simulink model "EPA_Walker"  (R2018a)
settings: Solver=FixedStepDiscrete  StartTime=0.0  StopTime=inf  FixedStep=0.001  RelTol=1e-3  EnableMultiTasking=on
model workspace (MAT data in the model file):
  MCOS : class17 (value not decoded)
undefined symbols (not defined in the file or in its folder): bits_current, bits_GRF, bits_Kd, bits_Kp, bits_position, bits_velocity, deadzone_in_TIB, deadzone_out_TIB, GRF_MAX, GRF_MIN, k_p_TIB, KD_MAX, KD_MIN, KP_MAX, KP_MIN, P_MAX, P_MIN, PressureFilter_CutOffFreq, PressureFilter_Gain, ReadingVoltage, T_MAX, T_MIN, V_MAX, V_MIN, voltageBias_GAS, voltageBias_GL, voltageBias_HAM, voltageBias_IL, voltageBias_POP, voltageBias_RF, voltageBias_SOL, voltageBias_TIB, voltageBias_VAS, voltageMultiplier_GAS, voltageMultiplier_GL, voltageMultiplier_HAM, voltageMultiplier_IL, voltageMultiplier_POP, voltageMultiplier_RF, voltageMultiplier_SOL, voltageMultiplier_TIB, voltageMultiplier_VAS, VoltageResolution
libraries: xpcethercatlib x139, simulink x19, peGeneralControl x18, slrtlib x9
(part 4 of 5)

== system EPA_Walker/PAMs/PAMs Right/IL ==
  Pressure Des : Inport
  Delay : Delay  DelayLength=1
  PID Controller : simulink/Continuous/PID Controller  Controller=PID  TimeDomain=Discrete-time  SampleTime=-1  IntegratorMethod=Forward Euler  FilterMethod=Forward Euler  Form=Ideal  UseFilter=on  ControllerParametersSource=external  P=k_p_pam  I=0  D=0.45*0.15/8  N=100  InitialConditionSource=internal  InitialConditionForIntegrator=0  InitialConditionForFilter=0  ExternalReset=none  LimitOutput=off  UpperSaturationLimit=inf  LowerSaturationLimit=-inf  LinearizeAsGain=on  AntiWindupMode=none  Kb=1  TrackingMode=off  Kt=1  PParamMin=[]  PParamMax=[]  IParamMin=[]  IParamMax=[]  DParamMin=[]  DParamMax=[]  NParamMin=[]  NParamMax=[]  KbParamMin=[]  KbParamMax=[]  KtParamMin=[]  KtParamMax=[]  POutMin=[]  POutMax=[]  IOutMin=[]  IOutMax=[]  DOutMin=[]  DOutMax=[]  NOutMin=[]  NOutMax=[]  KbOutMin=[]  KbOutMax=[]  KtOutMin=[]  KtOutMax=[]  IntegratorOutMin=[]  IntegratorOutMax=[]  FilterOutMin=[]  FilterOutMax=[]  SumOutMin=[]  SumOutMax=[]  SumI1OutMin=[]  SumI1OutMax=[]  SumI2OutMin=[]  SumI2OutMax=[]  SumI3OutMin=[]  SumI3OutMax=[]  SumDOutMin=[]  SumDOutMax=[]  SaturationOutMin=[]  SaturationOutMax=[]  IntegratorContinuousStateAttributes=''  IntegratorStateMustResolveToSignalObject=off  IntegratorRTWStateStorageClass=Auto  FilterContinuousStateAttributes=''  FilterStateMustResolveToSignalObject=off  FilterRTWStateStorageClass=Auto  DifferentiatorICPrevScaledInput=0  DifferentiatorOutMin=[]  DifferentiatorOutMax=[]  FilterDiffOutCoefMin=[]  FilterDiffOutCoefMax=[]  SumDenOutMin=[]  SumDenOutMax=[]  SumNumOutMin=[]  SumNumOutMax=[]  ReciprocalOutMin=[]  ReciprocalOutMax=[]  DivideOutMin=[]  DivideOutMax=[]  TunerSelectOption=Transfer Function Based (PID Tuner App)
  Solenoids : MATLAB Function  TreatAsAtomicUnit=on
  Sum : Sum  Inputs=|+-
  tag scope: R_IL_in=global, R_IL_out=global
  wires:
  Solenoids/3(inside_deadzone_1) -> Delay/1
  Delay/1 -> Solenoids/2(inside_deadzone)
  Pressure Des/1 -> Sum/1
  [R_IL_pres] -> Sum/2
  [R_deadzone_in] -> Solenoids/3(deadzone_in)
  [R_deadzone_out] -> Solenoids/4(deadzone_out)
  Solenoids/1(intake) -> [R_IL_in]
  Solenoids/2(outtake) -> [R_IL_out]
  [R_k_i] -> PID Controller/3
  [R_k_d] -> PID Controller/4
  [R_N] -> PID Controller/5
  Sum/1 -> PID Controller/1
  PID Controller/1 -> Solenoids/1(control)
  [R_k_p] -> PID Controller/2
  [R_PAMs_off] -> Solenoids/5(PAMs_on)
  [System_on] -> Solenoids/6(System_on)
  [R_Depressurize_PAMs] -> Solenoids/7(depressurize)

== system EPA_Walker/PAMs/PAMs Right/POP ==
  Pressure Des : Inport
  Delay : Delay  DelayLength=1
  PID Controller : simulink/Continuous/PID Controller  Controller=PID  TimeDomain=Discrete-time  SampleTime=-1  IntegratorMethod=Forward Euler  FilterMethod=Forward Euler  Form=Ideal  UseFilter=on  ControllerParametersSource=external  P=k_p_pam  I=0  D=0.45*0.15/8  N=100  InitialConditionSource=internal  InitialConditionForIntegrator=0  InitialConditionForFilter=0  ExternalReset=none  LimitOutput=off  UpperSaturationLimit=inf  LowerSaturationLimit=-inf  LinearizeAsGain=on  AntiWindupMode=none  Kb=1  TrackingMode=off  Kt=1  PParamMin=[]  PParamMax=[]  IParamMin=[]  IParamMax=[]  DParamMin=[]  DParamMax=[]  NParamMin=[]  NParamMax=[]  KbParamMin=[]  KbParamMax=[]  KtParamMin=[]  KtParamMax=[]  POutMin=[]  POutMax=[]  IOutMin=[]  IOutMax=[]  DOutMin=[]  DOutMax=[]  NOutMin=[]  NOutMax=[]  KbOutMin=[]  KbOutMax=[]  KtOutMin=[]  KtOutMax=[]  IntegratorOutMin=[]  IntegratorOutMax=[]  FilterOutMin=[]  FilterOutMax=[]  SumOutMin=[]  SumOutMax=[]  SumI1OutMin=[]  SumI1OutMax=[]  SumI2OutMin=[]  SumI2OutMax=[]  SumI3OutMin=[]  SumI3OutMax=[]  SumDOutMin=[]  SumDOutMax=[]  SaturationOutMin=[]  SaturationOutMax=[]  IntegratorContinuousStateAttributes=''  IntegratorStateMustResolveToSignalObject=off  IntegratorRTWStateStorageClass=Auto  FilterContinuousStateAttributes=''  FilterStateMustResolveToSignalObject=off  FilterRTWStateStorageClass=Auto  DifferentiatorICPrevScaledInput=0  DifferentiatorOutMin=[]  DifferentiatorOutMax=[]  FilterDiffOutCoefMin=[]  FilterDiffOutCoefMax=[]  SumDenOutMin=[]  SumDenOutMax=[]  SumNumOutMin=[]  SumNumOutMax=[]  ReciprocalOutMin=[]  ReciprocalOutMax=[]  DivideOutMin=[]  DivideOutMax=[]  TunerSelectOption=Transfer Function Based (PID Tuner App)
  Solenoids : MATLAB Function  TreatAsAtomicUnit=on
  Sum : Sum  Inputs=|+-
  tag scope: R_POP_in=global, R_POP_out=global
  wires:
  Solenoids/3(inside_deadzone_1) -> Delay/1
  Delay/1 -> Solenoids/2(inside_deadzone)
  Pressure Des/1 -> Sum/1
  [R_POP_pres] -> Sum/2
  [R_deadzone_in_pop] -> Solenoids/3(deadzone_in)
  [R_deadzone_out_pop] -> Solenoids/4(deadzone_out)
  Solenoids/1(intake) -> [R_POP_in]
  Solenoids/2(outtake) -> [R_POP_out]
  [R_k_i] -> PID Controller/3
  [R_k_d] -> PID Controller/4
  [R_N] -> PID Controller/5
  Sum/1 -> PID Controller/1
  PID Controller/1 -> Solenoids/1(control)
  [R_k_p] -> PID Controller/2
  [R_PAMs_off] -> Solenoids/5(PAMs_on)
  [System_on] -> Solenoids/6(System_on)
  [R_Depressurize_PAMs] -> Solenoids/7(depressurize)

== system EPA_Walker/PAMs/PAMs Right/RF ==
  Pressure Des : Inport
  Delay : Delay  DelayLength=1
  PID Controller : simulink/Continuous/PID Controller  Controller=PID  TimeDomain=Discrete-time  SampleTime=-1  IntegratorMethod=Forward Euler  FilterMethod=Forward Euler  Form=Ideal  UseFilter=on  ControllerParametersSource=external  P=k_p_pam  I=0  D=0.45*0.15/8  N=100  InitialConditionSource=internal  InitialConditionForIntegrator=0  InitialConditionForFilter=0  ExternalReset=none  LimitOutput=off  UpperSaturationLimit=inf  LowerSaturationLimit=-inf  LinearizeAsGain=on  AntiWindupMode=none  Kb=1  TrackingMode=off  Kt=1  PParamMin=[]  PParamMax=[]  IParamMin=[]  IParamMax=[]  DParamMin=[]  DParamMax=[]  NParamMin=[]  NParamMax=[]  KbParamMin=[]  KbParamMax=[]  KtParamMin=[]  KtParamMax=[]  POutMin=[]  POutMax=[]  IOutMin=[]  IOutMax=[]  DOutMin=[]  DOutMax=[]  NOutMin=[]  NOutMax=[]  KbOutMin=[]  KbOutMax=[]  KtOutMin=[]  KtOutMax=[]  IntegratorOutMin=[]  IntegratorOutMax=[]  FilterOutMin=[]  FilterOutMax=[]  SumOutMin=[]  SumOutMax=[]  SumI1OutMin=[]  SumI1OutMax=[]  SumI2OutMin=[]  SumI2OutMax=[]  SumI3OutMin=[]  SumI3OutMax=[]  SumDOutMin=[]  SumDOutMax=[]  SaturationOutMin=[]  SaturationOutMax=[]  IntegratorContinuousStateAttributes=''  IntegratorStateMustResolveToSignalObject=off  IntegratorRTWStateStorageClass=Auto  FilterContinuousStateAttributes=''  FilterStateMustResolveToSignalObject=off  FilterRTWStateStorageClass=Auto  DifferentiatorICPrevScaledInput=0  DifferentiatorOutMin=[]  DifferentiatorOutMax=[]  FilterDiffOutCoefMin=[]  FilterDiffOutCoefMax=[]  SumDenOutMin=[]  SumDenOutMax=[]  SumNumOutMin=[]  SumNumOutMax=[]  ReciprocalOutMin=[]  ReciprocalOutMax=[]  DivideOutMin=[]  DivideOutMax=[]  TunerSelectOption=Transfer Function Based (PID Tuner App)
  Solenoids : MATLAB Function  TreatAsAtomicUnit=on
  Sum : Sum  Inputs=|+-
  tag scope: R_RF_in=global, R_RF_out=global
  wires:
  Solenoids/3(inside_deadzone_1) -> Delay/1
  Delay/1 -> Solenoids/2(inside_deadzone)
  Pressure Des/1 -> Sum/1
  [R_RF_pres] -> Sum/2
  [R_deadzone_in] -> Solenoids/3(deadzone_in)
  [R_deadzone_out] -> Solenoids/4(deadzone_out)
  Solenoids/1(intake) -> [R_RF_in]
  Solenoids/2(outtake) -> [R_RF_out]
  [R_k_i] -> PID Controller/3
  [R_k_d] -> PID Controller/4
  [R_N] -> PID Controller/5
  Sum/1 -> PID Controller/1
  PID Controller/1 -> Solenoids/1(control)
  [R_k_p] -> PID Controller/2
  [R_PAMs_off] -> Solenoids/5(PAMs_on)
  [System_on] -> Solenoids/6(System_on)
  [R_Depressurize_PAMs] -> Solenoids/7(depressurize)

== system EPA_Walker/PAMs/PAMs Right/SOL ==
  Pressure Des : Inport
  Delay : Delay  DelayLength=1
  PID Controller : simulink/Continuous/PID Controller  Controller=PID  TimeDomain=Discrete-time  SampleTime=-1  IntegratorMethod=Forward Euler  FilterMethod=Forward Euler  Form=Ideal  UseFilter=on  ControllerParametersSource=external  P=k_p_pam  I=0  D=0.45*0.15/8  N=100  InitialConditionSource=internal  InitialConditionForIntegrator=0  InitialConditionForFilter=0  ExternalReset=none  LimitOutput=off  UpperSaturationLimit=inf  LowerSaturationLimit=-inf  LinearizeAsGain=on  AntiWindupMode=none  Kb=1  TrackingMode=off  Kt=1  PParamMin=[]  PParamMax=[]  IParamMin=[]  IParamMax=[]  DParamMin=[]  DParamMax=[]  NParamMin=[]  NParamMax=[]  KbParamMin=[]  KbParamMax=[]  KtParamMin=[]  KtParamMax=[]  POutMin=[]  POutMax=[]  IOutMin=[]  IOutMax=[]  DOutMin=[]  DOutMax=[]  NOutMin=[]  NOutMax=[]  KbOutMin=[]  KbOutMax=[]  KtOutMin=[]  KtOutMax=[]  IntegratorOutMin=[]  IntegratorOutMax=[]  FilterOutMin=[]  FilterOutMax=[]  SumOutMin=[]  SumOutMax=[]  SumI1OutMin=[]  SumI1OutMax=[]  SumI2OutMin=[]  SumI2OutMax=[]  SumI3OutMin=[]  SumI3OutMax=[]  SumDOutMin=[]  SumDOutMax=[]  SaturationOutMin=[]  SaturationOutMax=[]  IntegratorContinuousStateAttributes=''  IntegratorStateMustResolveToSignalObject=off  IntegratorRTWStateStorageClass=Auto  FilterContinuousStateAttributes=''  FilterStateMustResolveToSignalObject=off  FilterRTWStateStorageClass=Auto  DifferentiatorICPrevScaledInput=0  DifferentiatorOutMin=[]  DifferentiatorOutMax=[]  FilterDiffOutCoefMin=[]  FilterDiffOutCoefMax=[]  SumDenOutMin=[]  SumDenOutMax=[]  SumNumOutMin=[]  SumNumOutMax=[]  ReciprocalOutMin=[]  ReciprocalOutMax=[]  DivideOutMin=[]  DivideOutMax=[]  TunerSelectOption=Transfer Function Based (PID Tuner App)
  Solenoids : MATLAB Function  TreatAsAtomicUnit=on
  Sum : Sum  Inputs=|+-
  tag scope: R_SOL_in=global, R_SOL_out=global
  wires:
  Solenoids/3(inside_deadzone_1) -> Delay/1
  Delay/1 -> Solenoids/2(inside_deadzone)
  PID Controller/1 -> Solenoids/1(control)
  Pressure Des/1 -> Sum/1
  [R_SOL_pres] -> Sum/2
  [R_deadzone_in] -> Solenoids/3(deadzone_in)
  [R_deadzone_out] -> Solenoids/4(deadzone_out)
  Solenoids/1(intake) -> [R_SOL_in]
  Solenoids/2(outtake) -> [R_SOL_out]
  [R_k_i] -> PID Controller/3
  [R_k_d] -> PID Controller/4
  [R_N] -> PID Controller/5
  Sum/1 -> PID Controller/1
  [R_k_p] -> PID Controller/2
  [R_PAMs_off] -> Solenoids/5(PAMs_on)
  [System_on] -> Solenoids/6(System_on)
  [R_Depressurize_PAMs] -> Solenoids/7(depressurize)

== system EPA_Walker/PAMs/PAMs Right/TIB ==
  Pressure Des : Inport
  Delay : Delay  DelayLength=1
  PID Controller : simulink/Continuous/PID Controller  Controller=PID  TimeDomain=Discrete-time  SampleTime=-1  IntegratorMethod=Forward Euler  FilterMethod=Forward Euler  Form=Ideal  UseFilter=on  ControllerParametersSource=internal  P=k_p_TIB  I=0  D=0.01  N=300  InitialConditionSource=internal  InitialConditionForIntegrator=0  InitialConditionForFilter=0  ExternalReset=none  LimitOutput=off  UpperSaturationLimit=inf  LowerSaturationLimit=-inf  LinearizeAsGain=on  AntiWindupMode=none  Kb=1  TrackingMode=off  Kt=1  PParamMin=[]  PParamMax=[]  IParamMin=[]  IParamMax=[]  DParamMin=[]  DParamMax=[]  NParamMin=[]  NParamMax=[]  KbParamMin=[]  KbParamMax=[]  KtParamMin=[]  KtParamMax=[]  POutMin=[]  POutMax=[]  IOutMin=[]  IOutMax=[]  DOutMin=[]  DOutMax=[]  NOutMin=[]  NOutMax=[]  KbOutMin=[]  KbOutMax=[]  KtOutMin=[]  KtOutMax=[]  IntegratorOutMin=[]  IntegratorOutMax=[]  FilterOutMin=[]  FilterOutMax=[]  SumOutMin=[]  SumOutMax=[]  SumI1OutMin=[]  SumI1OutMax=[]  SumI2OutMin=[]  SumI2OutMax=[]  SumI3OutMin=[]  SumI3OutMax=[]  SumDOutMin=[]  SumDOutMax=[]  SaturationOutMin=[]  SaturationOutMax=[]  IntegratorContinuousStateAttributes=''  IntegratorStateMustResolveToSignalObject=off  IntegratorRTWStateStorageClass=Auto  FilterContinuousStateAttributes=''  FilterStateMustResolveToSignalObject=off  FilterRTWStateStorageClass=Auto  DifferentiatorICPrevScaledInput=0  DifferentiatorOutMin=[]  DifferentiatorOutMax=[]  FilterDiffOutCoefMin=[]  FilterDiffOutCoefMax=[]  SumDenOutMin=[]  SumDenOutMax=[]  SumNumOutMin=[]  SumNumOutMax=[]  ReciprocalOutMin=[]  ReciprocalOutMax=[]  DivideOutMin=[]  DivideOutMax=[]  TunerSelectOption=Transfer Function Based (PID Tuner App)
  Solenoids : MATLAB Function  TreatAsAtomicUnit=on
  Sum : Sum  Inputs=|+-
  tag scope: R_TIB_in=global, R_TIB_out=global
  wires:
  Solenoids/3(inside_deadzone_1) -> Delay/1
  Delay/1 -> Solenoids/2(inside_deadzone)
  Pressure Des/1 -> Sum/1
  [R_TIB_pres] -> Sum/2
  Solenoids/1(intake) -> [R_TIB_in]
  Solenoids/2(outtake) -> [R_TIB_out]
  [R_PAMs_off] -> Solenoids/3(PAMs_on)
  [System_on] -> Solenoids/4(System_on)
  PID Controller/1 -> Solenoids/1(control)
  Sum/1 -> PID Controller/1
  [R_Depressurize_PAMs] -> Solenoids/5(depressurize)

== system EPA_Walker/PAMs/PAMs Right/VAS ==
  Pressure Des : Inport
  Delay : Delay  DelayLength=1
  PID Controller : simulink/Continuous/PID Controller  Controller=PID  TimeDomain=Discrete-time  SampleTime=-1  IntegratorMethod=Forward Euler  FilterMethod=Forward Euler  Form=Ideal  UseFilter=on  ControllerParametersSource=external  P=k_p_pam  I=0  D=0.45*0.15/8  N=100  InitialConditionSource=internal  InitialConditionForIntegrator=0  InitialConditionForFilter=0  ExternalReset=none  LimitOutput=off  UpperSaturationLimit=inf  LowerSaturationLimit=-inf  LinearizeAsGain=on  AntiWindupMode=none  Kb=1  TrackingMode=off  Kt=1  PParamMin=[]  PParamMax=[]  IParamMin=[]  IParamMax=[]  DParamMin=[]  DParamMax=[]  NParamMin=[]  NParamMax=[]  KbParamMin=[]  KbParamMax=[]  KtParamMin=[]  KtParamMax=[]  POutMin=[]  POutMax=[]  IOutMin=[]  IOutMax=[]  DOutMin=[]  DOutMax=[]  NOutMin=[]  NOutMax=[]  KbOutMin=[]  KbOutMax=[]  KtOutMin=[]  KtOutMax=[]  IntegratorOutMin=[]  IntegratorOutMax=[]  FilterOutMin=[]  FilterOutMax=[]  SumOutMin=[]  SumOutMax=[]  SumI1OutMin=[]  SumI1OutMax=[]  SumI2OutMin=[]  SumI2OutMax=[]  SumI3OutMin=[]  SumI3OutMax=[]  SumDOutMin=[]  SumDOutMax=[]  SaturationOutMin=[]  SaturationOutMax=[]  IntegratorContinuousStateAttributes=''  IntegratorStateMustResolveToSignalObject=off  IntegratorRTWStateStorageClass=Auto  FilterContinuousStateAttributes=''  FilterStateMustResolveToSignalObject=off  FilterRTWStateStorageClass=Auto  DifferentiatorICPrevScaledInput=0  DifferentiatorOutMin=[]  DifferentiatorOutMax=[]  FilterDiffOutCoefMin=[]  FilterDiffOutCoefMax=[]  SumDenOutMin=[]  SumDenOutMax=[]  SumNumOutMin=[]  SumNumOutMax=[]  ReciprocalOutMin=[]  ReciprocalOutMax=[]  DivideOutMin=[]  DivideOutMax=[]  TunerSelectOption=Transfer Function Based (PID Tuner App)
  Solenoids : MATLAB Function  TreatAsAtomicUnit=on
  Sum : Sum  Inputs=|+-
  tag scope: R_VAS_in=global, R_VAS_out=global
  wires:
  Solenoids/3(inside_deadzone_1) -> Delay/1
  Delay/1 -> Solenoids/2(inside_deadzone)
  Pressure Des/1 -> Sum/1
  [R_VAS_pres] -> Sum/2
  [R_deadzone_in] -> Solenoids/3(deadzone_in)
  [R_deadzone_out] -> Solenoids/4(deadzone_out)
  Solenoids/1(intake) -> [R_VAS_in]
  [R_k_i] -> PID Controller/3
  [R_k_d] -> PID Controller/4
  [R_N] -> PID Controller/5
  Sum/1 -> PID Controller/1
  PID Controller/1 -> Solenoids/1(control)
  [R_k_p] -> PID Controller/2
  [R_PAMs_off] -> Solenoids/5(PAMs_on)
  [System_on] -> Solenoids/6(System_on)
  Solenoids/2(outtake) -> [R_VAS_out]
  [R_Depressurize_PAMs] -> Solenoids/7(depressurize)

== system EPA_Walker/Ethernet Communication/Inputs/GRF Slave/GRFx  ==
  Data Type Conversion3 : DataTypeConversion
  EtherCAT PDO Receive21 : xpcethercatlib/EtherCAT PDO Receive  Priority=2  sig_name=GRF.Inputs.Byte0  sig_offset=0  sig_type=uint8  type_size=8  sig_dim=1  device_id=0  sample_time=0.001000
      settings: SourceProductName=Simulink Real-Time  SourceProductBaseCode=XP
  EtherCAT PDO Receive22 : xpcethercatlib/EtherCAT PDO Receive  Priority=2  sig_name=GRF.Inputs.Byte1  sig_offset=8  sig_type=uint8  type_size=8  sig_dim=1  device_id=0  sample_time=0.001000
      settings: SourceProductName=Simulink Real-Time  SourceProductBaseCode=XP
  Gain24 : Gain  Gain=256
  Hip Position Transformation : MATLAB Function  TreatAsAtomicUnit=on
  Sum5 : Sum
  tag scope: GRFx_Volts=global
  wires:
  EtherCAT PDO Receive21/1 -> Gain24/1
  Hip Position Transformation/1(GRF_x) -> [GRFx_Volts]
  Sum5/1 -> Data Type Conversion3/1
  EtherCAT PDO Receive22/1 -> Sum5/2
  Gain24/1 -> Sum5/1
  Data Type Conversion3/1 -> Hip Position Transformation/1(x_int)

== system EPA_Walker/Ethernet Communication/Inputs/GRF Slave/GRFy  ==
  Data Type Conversion3 : DataTypeConversion
  EtherCAT PDO Receive21 : xpcethercatlib/EtherCAT PDO Receive  Priority=2  sig_name=GRF.Inputs.Byte2  sig_offset=16  sig_type=uint8  type_size=8  sig_dim=1  device_id=0  sample_time=0.001000
      settings: SourceProductName=Simulink Real-Time  SourceProductBaseCode=XP
  EtherCAT PDO Receive22 : xpcethercatlib/EtherCAT PDO Receive  Priority=2  sig_name=GRF.Inputs.Byte3  sig_offset=24  sig_type=uint8  type_size=8  sig_dim=1  device_id=0  sample_time=0.001000
      settings: SourceProductName=Simulink Real-Time  SourceProductBaseCode=XP
  Gain24 : Gain  Gain=256
  Hip Position Transformation : MATLAB Function  TreatAsAtomicUnit=on
  Sum5 : Sum
  tag scope: GRFy_Volts=global
  wires:
  EtherCAT PDO Receive21/1 -> Gain24/1
  Hip Position Transformation/1(GRF_y) -> [GRFy_Volts]
  Sum5/1 -> Data Type Conversion3/1
  EtherCAT PDO Receive22/1 -> Sum5/2
  Gain24/1 -> Sum5/1
  Data Type Conversion3/1 -> Hip Position Transformation/1(x_int)

== system EPA_Walker/Ethernet Communication/Inputs/GRF Slave/GRFz  ==
  Data Type Conversion3 : DataTypeConversion
  EtherCAT PDO Receive21 : xpcethercatlib/EtherCAT PDO Receive  Priority=2  sig_name=GRF.Inputs.Byte4  sig_offset=32  sig_type=uint8  type_size=8  sig_dim=1  device_id=0  sample_time=0.001000
      settings: SourceProductName=Simulink Real-Time  SourceProductBaseCode=XP
  EtherCAT PDO Receive22 : xpcethercatlib/EtherCAT PDO Receive  Priority=2  sig_name=GRF.Inputs.Byte5  sig_offset=40  sig_type=uint8  type_size=8  sig_dim=1  device_id=0  sample_time=0.001000
      settings: SourceProductName=Simulink Real-Time  SourceProductBaseCode=XP
  Gain24 : Gain  Gain=256
  Hip Position Transformation : MATLAB Function  TreatAsAtomicUnit=on
  Sum5 : Sum
  tag scope: GRFz_Volts=global
  wires:
  Sum5/1 -> Data Type Conversion3/1
  Hip Position Transformation/1(GRF_z) -> [GRFz_Volts]
  EtherCAT PDO Receive21/1 -> Gain24/1
  Gain24/1 -> Sum5/1
  EtherCAT PDO Receive22/1 -> Sum5/2
  Data Type Conversion3/1 -> Hip Position Transformation/1(x_int)

== system EPA_Walker/High Level Control/HL Left/Stance phase/FMCH (Static) ==
  GRF_Z : Inport
  angHip : Inport  Port=2
  C_Hip : Inport  Port=3
  Phi_0_Hip : Inport  Port=4
  Add1 : Sum  Inputs=+-
  Gain2 : Gain
  Gain3 : Gain  Gain=pi/180
  Multiply1 : Product
  Multiply2 : Product
  torMotHip : Outport  InitialOutput=0
  wires:
  Add1/1 -> Gain3/1
  GRF_Z/1 -> Multiply1/1
  Multiply1/1 -> Multiply2/2
  angHip/1 -> Add1/1
  Multiply2/1 -> Gain2/1
  Phi_0_Hip/1 -> Add1/2
  C_Hip/1 -> Multiply2/1
  Gain2/1 -> torMotHip/1
  Gain3/1 -> Multiply1/2

== system EPA_Walker/High Level Control/HL Left/Stance phase/FMCK (Static) ==
  GRF_Z : Inport
  angKne : Inport  Port=2
  C_ : Inport  Port=3
  Phi_0 : Inport  Port=4
  Add1 : Sum  Inputs=+-
  Gain2 : Gain
  Gain3 : Gain  Gain=pi/180
  Multiply1 : Product
  Multiply2 : Product
  torMotKne : Outport  InitialOutput=0
  wires:
  Add1/1 -> Gain3/1
  GRF_Z/1 -> Multiply1/1
  Multiply1/1 -> Multiply2/2
  angKne/1 -> Add1/1
  Multiply2/1 -> Gain2/1
  Phi_0/1 -> Add1/2
  C_/1 -> Multiply2/1
  Gain2/1 -> torMotKne/1
  Gain3/1 -> Multiply1/2

== system EPA_Walker/High Level Control/HL Right/Stance phase/FMCH (Static) ==
  GRF_Z : Inport
  angHip : Inport  Port=2
  C_Hip : Inport  Port=3
  Phi_0_Hip : Inport  Port=4
  Add1 : Sum  Inputs=+-
  Gain2 : Gain
  Gain3 : Gain  Gain=pi/180
  Multiply1 : Product
  Multiply2 : Product
  torMotHip : Outport  InitialOutput=0
  wires:
  Add1/1 -> Gain3/1
  GRF_Z/1 -> Multiply1/1
  Multiply1/1 -> Multiply2/2
  angHip/1 -> Add1/1
  Multiply2/1 -> Gain2/1
  Phi_0_Hip/1 -> Add1/2
  C_Hip/1 -> Multiply2/1
  Gain2/1 -> torMotHip/1
  Gain3/1 -> Multiply1/2

== system EPA_Walker/High Level Control/HL Right/Stance phase/FMCK (Static) ==
  GRF_Z : Inport
  angKne : Inport  Port=2
  C_ : Inport  Port=3
  Phi_0 : Inport  Port=4
  Add1 : Sum  Inputs=+-
  Gain2 : Gain
  Gain3 : Gain  Gain=pi/180
  Multiply1 : Product
  Multiply2 : Product
  torMotKne : Outport  InitialOutput=0
  wires:
  Add1/1 -> Gain3/1
  GRF_Z/1 -> Multiply1/1
  Multiply1/1 -> Multiply2/2
  angKne/1 -> Add1/1
  Multiply2/1 -> Gain2/1
  Phi_0/1 -> Add1/2
  C_/1 -> Multiply2/1
  Gain2/1 -> torMotKne/1
  Gain3/1 -> Multiply1/2

== matlab function EPA_Walker/Ethernet Communication/Inputs/Motor Left/Byte Splitting Knee ==
  data: byte input; Vel_low output; Curr_h output
function [Vel_low,Curr_h] = fcn(byte)

Vel_low = bitshift(byte,-4);
Curr_h = bitand(byte,15);

== matlab function EPA_Walker/Safety /System On/Emergency Switch ==
  data: Emergency_switch input; y output
function y = fcn(Emergency_switch)

if Emergency_switch >= 3500
    y = 1;
else
    y = 0;
end

== matlab function EPA_Walker/Ethernet Communication/Inputs/Motor Left/Byte Splitting Hip ==
  data: byte input; Vel_low output; Curr_h output
function [Vel_low,Curr_h] = fcn(byte)

Vel_low = bitshift(byte,-4);
Curr_h = bitand(byte,15);

== matlab function EPA_Walker/Ethernet Communication/Inputs/Motor Left/Hip Position Transformation ==
  data: x_int input; Hip_position output; P_MIN parameter; P_MAX parameter; bits_position parameter
function Hip_position = uint_to_float(x_int, P_MIN, P_MAX, bits_position)
    Hip_position = uint_to_float(x_int, P_MIN, P_MAX, bits_position);
end

== matlab function EPA_Walker/Ethernet Communication/Inputs/Motor Left/Knee Position Transformation1 ==
  data: x_int input; Knee_position output; P_MIN parameter; P_MAX parameter; bits_position parameter
function Knee_position = uint_to_float(x_int, P_MIN, P_MAX, bits_position)
    Knee_position = uint_to_float(x_int, P_MIN, P_MAX, bits_position);
end

== matlab function EPA_Walker/Ethernet Communication/Inputs/Motor Left/Hip Velocity Transformation ==
  data: x_int input; Hip_velocity output; V_MIN parameter; V_MAX parameter; bits_velocity parameter
function Hip_velocity = uint_to_float(x_int, V_MIN, V_MAX, bits_velocity)
    % Converts an unsigned int to float, given range and number of bits %
    Hip_velocity = uint_to_float(x_int, V_MIN, V_MAX, bits_velocity);

end

== matlab function EPA_Walker/Ethernet Communication/Inputs/Motor Left/Hip Current Transformation ==
  data: x_int input; Hip_current output; T_MIN parameter; T_MAX parameter; bits_current parameter
function Hip_current = uint_to_float(x_int, T_MIN, T_MAX, bits_current)
    % Converts an unsigned int to float, given range and number of bits %
    Hip_current = uint_to_float(x_int, T_MIN, T_MAX, bits_current);
end

== matlab function EPA_Walker/Ethernet Communication/Inputs/Motor Left/Knee Velocity Transformation1 ==
  data: x_int input; Knee_velocity output; V_MIN parameter; V_MAX parameter; bits_velocity parameter
function Knee_velocity = uint_to_float(x_int, V_MIN, V_MAX, bits_velocity)
    Knee_velocity = uint_to_float(x_int, V_MIN, V_MAX, bits_velocity);
end

== matlab function EPA_Walker/Ethernet Communication/Inputs/Motor Left/Knee Current Tranformation ==
  data: x_int input; Knee_current output; T_MIN parameter; T_MAX parameter; bits_current parameter
function Knee_current = uint_to_float(x_int, T_MIN, T_MAX, bits_current)
    Knee_current = uint_to_float(x_int, T_MIN, T_MAX, bits_current);
end

== matlab function EPA_Walker/Ethernet Communication/Outputs/Motor Left/MATLAB Function ==
  data: x input; x_int output; P_MIN parameter; P_MAX parameter; bits_position parameter
function x_int = float_to_uint(x, P_MIN, P_MAX, bits_position)
    % Converts a float to an unsigned int, given range and number of bits_position %
    x_int = float_to_uint(x, P_MIN, P_MAX, bits_position);
end

== matlab function EPA_Walker/Ethernet Communication/Outputs/Motor Left/Byte Splitting Position ==
  data: byte input; Pos_h output; Pos_l output
function [Pos_h,Pos_l] = fcn(byte)

Pos_l = bitand(byte,255);
Pos_h = bitshift(byte,-8);

== matlab function EPA_Walker/Ethernet Communication/Outputs/Motor Left/Byte Splitting Position1 ==
  data: byte input; Vel_h output; Vel_l output
function [Vel_h,Vel_l] = fcn(byte)

Vel_l = bitand(byte,15);
Vel_h = bitshift(byte,-4);

== matlab function EPA_Walker/Ethernet Communication/Outputs/Motor Left/MATLAB Function1 ==
  data: x input; x_int output; V_MIN parameter; V_MAX parameter; bits_velocity parameter
function x_int = float_to_uint(x, V_MIN, V_MAX, bits_velocity)
    % Converts a float to an unsigned int, given range and number of bits_velocity %
    x_int = float_to_uint(x, V_MIN, V_MAX, bits_velocity);
end

== matlab function EPA_Walker/Ethernet Communication/Outputs/Motor Left/Byte Splitting Position2 ==
  data: byte input; Kp_h output; Kp_l output
 function [Kp_h,Kp_l] = fcn(byte)

Kp_l = bitand(byte,255);
Kp_h = bitshift(byte,-8);

== matlab function EPA_Walker/Ethernet Communication/Outputs/Motor Left/MATLAB Function2 ==
  data: x input; x_int output; KP_MIN parameter; KP_MAX parameter; bits_Kp parameter
function x_int = float_to_uint(x, KP_MIN, KP_MAX, bits_Kp)
    % Converts a float to an unsigned int, given range and number of bits_Kp %
    x_int = float_to_uint(x, KP_MIN, KP_MAX, bits_Kp);

end

== matlab function EPA_Walker/Ethernet Communication/Outputs/Motor Left/Byte Splitting Position3 ==
  data: byte input; Kd_h output; Kd_l output
function [Kd_h,Kd_l] = fcn(byte)

Kd_l = bitand(byte,15);
Kd_h = bitshift(byte,-4);

== matlab function EPA_Walker/Ethernet Communication/Outputs/Motor Left/MATLAB Function3 ==
  data: x input; x_int output; KD_MIN parameter; KD_MAX parameter; bits_Kd parameter
function x_int = float_to_uint(x, KD_MIN, KD_MAX, bits_Kd)
    % Converts a float to an unsigned int, given range and number of bits_Kd %
    x_int = float_to_uint(x, KD_MIN, KD_MAX, bits_Kd);

end

== matlab function EPA_Walker/Ethernet Communication/Outputs/Motor Left/Byte Splitting Position4 ==
  data: byte input; Torque_h output; Torque_l output
function [Torque_h,Torque_l] = fcn(byte)

Torque_l = bitand(byte,255);
Torque_h = bitshift(byte,-8);

== matlab function EPA_Walker/Ethernet Communication/Outputs/Motor Left/MATLAB Function4 ==
  data: x input; x_int output; T_MIN parameter; T_MAX parameter; bits_current parameter
function x_int = float_to_uint(x, T_MIN, T_MAX, bits_current)
    % Converts a float to an unsigned int, given range and number of bits_current %
    x_int = float_to_uint(x, T_MIN, T_MAX, bits_current);

end

== matlab function EPA_Walker/Ethernet Communication/Outputs/Motor Left/Byte Splitting Position5 ==
  data: byte input; Pos_h output; Pos_l output
function [Pos_h,Pos_l] = fcn(byte)

Pos_l = bitand(byte,255);
Pos_h = bitshift(byte,-8);

== matlab function EPA_Walker/Ethernet Communication/Outputs/Motor Left/Byte Splitting Position6 ==
  data: byte input; Vel_h output; Vel_l output
function [Vel_h,Vel_l] = fcn(byte)

Vel_l = bitand(byte,15);
Vel_h = bitshift(byte,-4);

== matlab function EPA_Walker/Ethernet Communication/Outputs/Motor Left/Byte Splitting Position7 ==
  data: byte input; Kp_h output; Kp_l output
function [Kp_h,Kp_l] = fcn(byte)

Kp_l = bitand(byte,255);
Kp_h = bitshift(byte,-8);

== matlab function EPA_Walker/Ethernet Communication/Outputs/Motor Left/Byte Splitting Position8 ==
  data: byte input; Kd_h output; Kd_l output
function [Kd_h,Kd_l] = fcn(byte)

Kd_l = bitand(byte,15);
Kd_h = bitshift(byte,-4);

== matlab function EPA_Walker/Ethernet Communication/Outputs/Motor Left/Byte Splitting Position9 ==
  data: byte input; Torque_h output; Torque_l output
function [Torque_h,Torque_l] = fcn(byte)

Torque_l = bitand(byte,255);
Torque_h = bitshift(byte,-8);

== matlab function EPA_Walker/Ethernet Communication/Outputs/Motor Left/MATLAB Function5 ==
  data: x input; x_int output; P_MIN parameter; P_MAX parameter; bits_position parameter
function x_int = float_to_uint(x, P_MIN, P_MAX, bits_position)
    % Converts a float to an unsigned int, given range and number of bits_position %
    x_int = float_to_uint(x, P_MIN, P_MAX, bits_position);
end

== matlab function EPA_Walker/Ethernet Communication/Outputs/Motor Left/MATLAB Function6 ==
  data: x input; x_int output; V_MIN parameter; V_MAX parameter; bits_velocity parameter
function x_int = float_to_uint(x, V_MIN, V_MAX, bits_velocity)
    % Converts a float to an unsigned int, given range and number of bits_velocity %
    x_int = float_to_uint(x, V_MIN, V_MAX, bits_velocity);

end

== matlab function EPA_Walker/Ethernet Communication/Outputs/Motor Left/MATLAB Function7 ==
  data: x input; x_int output; KP_MIN parameter; KP_MAX parameter; bits_Kp parameter
function x_int = float_to_uint(x, KP_MIN, KP_MAX, bits_Kp)
    % Converts a float to an unsigned int, given range and number of bits_Kp %
    x_int = float_to_uint(x, KP_MIN, KP_MAX, bits_Kp);
end

== matlab function EPA_Walker/Ethernet Communication/Outputs/Motor Left/MATLAB Function8 ==
  data: x input; x_int output; KD_MIN parameter; KD_MAX parameter; bits_Kd parameter
function x_int = float_to_uint(x, KD_MIN, KD_MAX, bits_Kd)
    % Converts a float to an unsigned int, given range and number of bits_Kd %
    x_int = float_to_uint(x, KD_MIN, KD_MAX, bits_Kd);
end

== matlab function EPA_Walker/Ethernet Communication/Outputs/Motor Left/MATLAB Function9 ==
  data: x input; x_int output; T_MIN parameter; T_MAX parameter; bits_current parameter
function x_int = float_to_uint(x, T_MIN, T_MAX, bits_current)
    % Converts a float to an unsigned int, given range and number of bits_current %
    x_int = float_to_uint(x, T_MIN, T_MAX, bits_current);
end

== matlab function EPA_Walker/Motors/Motor Left/Motor Mode Handler ==
  data: Hip_Mode input; Hip_Mode_out output; Hip_position_des input; Hip_velocity_des input; Hip_Kp input; Hip_Kd input; Hip_Curret_des input; Hip_position_des_out output; Hip_velocity_des_out output; Hip_Kp_out output; Hip_Kd_out output; Hip_Curret_des_out output
function [Hip_Mode_out, Hip_position_des_out, Hip_velocity_des_out, Hip_Kp_out, Hip_Kd_out, Hip_Curret_des_out] = fcn(Hip_Mode, Hip_position_des, Hip_velocity_des, Hip_Kp, Hip_Kd, Hip_Curret_des)

[Hip_Mode_out, Hip_position_des_out, Hip_velocity_des_out, Hip_Kp_out, Hip_Kd_out, Hip_Curret_des_out] = Motor_handler(Hip_Mode, Hip_position_des, Hip_velocity_des, Hip_Kp, Hip_Kd, Hip_Curret_des);

end

== matlab function EPA_Walker/High Level Control/Walking Phase Detection ==
  data: GRFz input; isSwing output; previous_isSwing input
function isSwing = fcn(GRFz, previous_isSwing)
if GRFz > 10 && previous_isSwing == 1
    isSwing = 0;
elseif GRFz < 5 && previous_isSwing == 0 
    isSwing = 1;
else
    isSwing = previous_isSwing;
end

end

== matlab function EPA_Walker/Motors/Motor Left/Motor Mode Handler1 ==
  data: Knee_Mode input; Knee_Mode_out output; Knee_position_des input; Knee_velocity_des input; Knee_Kp input; Knee_Kd input; Knee_Curret_des input; Knee_position_des_out output; Knee_velocity_des_out output; Knee_Kp_out output; Knee_Kd_out output; Knee_Curret_des_out output
function [Knee_Mode_out, Knee_position_des_out, Knee_velocity_des_out, Knee_Kp_out, Knee_Kd_out, Knee_Curret_des_out] = fcn(Knee_Mode, Knee_position_des, Knee_velocity_des, Knee_Kp, Knee_Kd, Knee_Curret_des)

[Knee_Mode_out, Knee_position_des_out, Knee_velocity_des_out, Knee_Kp_out, Knee_Kd_out, Knee_Curret_des_out] = Motor_handler(Knee_Mode, Knee_position_des, Knee_velocity_des, Knee_Kp, Knee_Kd, Knee_Curret_des);

end

== matlab function EPA_Walker/Safety /MATLAB Function ==
  data: Hip_motor_safe output; Knee_motor_safe output; Motors_safe output; flag output; Hip_Position input; Knee_Position input; flag_1 input
function [Hip_motor_safe, Knee_motor_safe,Motors_safe,flag]= fcn(Hip_Position, Knee_Position, flag_1)

flag = flag_1;
if flag == 0
    if Hip_Position >= -50 && Hip_Position <50
        Hip_motor_safe = 1;
    else
        Hip_motor_safe = 0;   
        flag = 1;
    end
    if Knee_Position >= -10 && Knee_Position <110
        Knee_motor_safe = 1;
    else
        Knee_motor_safe = 0;  
        flag = 1;
    end
    Motors_safe = double(Hip_motor_safe & Knee_motor_safe);
else
    if Hip_Position >= -50 && Hip_Position <50
        Hip_motor_safe = 1;
    else
        Hip_motor_safe = 0;   
        flag = 1;
    end

    if Knee_Position >= -5 && Knee_Position <110
        Knee_motor_safe = 1;
    else
        Knee_motor_safe = 0;  
        flag = 1;
    end
    Motors_safe = 0;
end

end

== matlab function EPA_Walker/High Level Control/HL Left/Motor Modes ==
  data: isSwing input; Hip_mode output; Knee_mode output
function [Hip_mode, Knee_mode] = fcn(isSwing)

if isSwing == 1
    Hip_mode = 1;
    Knee_mode = 1;
elseif isSwing == 0
    Hip_mode = 2;
    Knee_mode = 2;
else
    Hip_mode = 0;
    Knee_mode = 0;
end
end

== matlab function EPA_Walker/Ethernet Communication/Inputs/PAMs Left/MATLAB Function ==
  data: sensorValue input; pressure output; voltageMultiplier_TIB parameter; voltageBias_TIB parameter; ReadingVoltage parameter; VoltageResolution parameter
function pressure   = fcn(sensorValue,voltageMultiplier_TIB, voltageBias_TIB,ReadingVoltage, VoltageResolution)
pressure   = PressureSensor(sensorValue,voltageMultiplier_TIB, voltageBias_TIB,ReadingVoltage,VoltageResolution);
end

== matlab function EPA_Walker/Ethernet Communication/Inputs/PAMs Left/MATLAB Function1 ==
  data: sensorValue input; pressure output; voltageMultiplier_SOL parameter; voltageBias_SOL parameter; ReadingVoltage parameter; VoltageResolution parameter
function pressure   = fcn(sensorValue,voltageMultiplier_SOL, voltageBias_SOL,ReadingVoltage, VoltageResolution)
pressure   = PressureSensor(sensorValue,voltageMultiplier_SOL, voltageBias_SOL,ReadingVoltage,VoltageResolution);
end

== matlab function EPA_Walker/Ethernet Communication/Inputs/PAMs Left/MATLAB Function2 ==
  data: sensorValue input; pressure output; voltageMultiplier_GAS parameter; voltageBias_GAS parameter; ReadingVoltage parameter; VoltageResolution parameter
function pressure   = fcn(sensorValue,voltageMultiplier_GAS, voltageBias_GAS,ReadingVoltage, VoltageResolution)
pressure   = PressureSensor(sensorValue,voltageMultiplier_GAS, voltageBias_GAS,ReadingVoltage,VoltageResolution);
end

== matlab function EPA_Walker/Ethernet Communication/Inputs/PAMs Left/MATLAB Function3 ==
  data: sensorValue input; pressure output; voltageMultiplier_VAS parameter; voltageBias_VAS parameter; ReadingVoltage parameter; VoltageResolution parameter
function pressure   = fcn(sensorValue,voltageMultiplier_VAS, voltageBias_VAS,ReadingVoltage, VoltageResolution)
pressure   = PressureSensor(sensorValue,voltageMultiplier_VAS, voltageBias_VAS,ReadingVoltage,VoltageResolution);
end

== matlab function EPA_Walker/Ethernet Communication/Inputs/PAMs Left/MATLAB Function4 ==
  data: sensorValue input; pressure output; voltageMultiplier_POP parameter; voltageBias_POP parameter; ReadingVoltage parameter; VoltageResolution parameter
function pressure   = fcn(sensorValue,voltageMultiplier_POP, voltageBias_POP,ReadingVoltage, VoltageResolution)
pressure   = PressureSensor(sensorValue,voltageMultiplier_POP, voltageBias_POP,ReadingVoltage,VoltageResolution);
end

== matlab function EPA_Walker/Ethernet Communication/Inputs/PAMs Left/MATLAB Function5 ==
  data: sensorValue input; pressure output; voltageMultiplier_RF parameter; voltageBias_RF parameter; ReadingVoltage parameter; VoltageResolution parameter
function pressure   = fcn(sensorValue,voltageMultiplier_RF, voltageBias_RF,ReadingVoltage, VoltageResolution)
pressure   = PressureSensor(sensorValue,voltageMultiplier_RF, voltageBias_RF,ReadingVoltage,VoltageResolution);
end

== matlab function EPA_Walker/Ethernet Communication/Inputs/PAMs Left/MATLAB Function6 ==
  data: sensorValue input; pressure output; voltageMultiplier_HAM parameter; voltageBias_HAM parameter; ReadingVoltage parameter; VoltageResolution parameter
function pressure   = fcn(sensorValue,voltageMultiplier_HAM, voltageBias_HAM,ReadingVoltage, VoltageResolution)
pressure   = PressureSensor(sensorValue,voltageMultiplier_HAM, voltageBias_HAM,ReadingVoltage,VoltageResolution);
end

== matlab function EPA_Walker/Ethernet Communication/Inputs/PAMs Left/MATLAB Function7 ==
  data: sensorValue input; pressure output; voltageMultiplier_IL parameter; voltageBias_IL parameter; ReadingVoltage parameter; VoltageResolution parameter
function pressure   = fcn(sensorValue,voltageMultiplier_IL, voltageBias_IL,ReadingVoltage, VoltageResolution)
pressure   = PressureSensor(sensorValue,voltageMultiplier_IL, voltageBias_IL,ReadingVoltage,VoltageResolution);
end

== matlab function EPA_Walker/Ethernet Communication/Inputs/PAMs Left/MATLAB Function8 ==
  data: sensorValue input; pressure output; voltageMultiplier_GL parameter; voltageBias_GL parameter; ReadingVoltage parameter; VoltageResolution parameter
function pressure   = fcn(sensorValue,voltageMultiplier_GL, voltageBias_GL,ReadingVoltage, VoltageResolution)
pressure   = PressureSensor(sensorValue,voltageMultiplier_GL, voltageBias_GL,ReadingVoltage,VoltageResolution);
end

== matlab function EPA_Walker/PAMs/PAMs Left/TIB/Solenoids ==
  data: control input; intake output; inside_deadzone input; outtake output; inside_deadzone_1 output; PAMs_on input; System_on input; deadzone_in_TIB parameter; deadzone_out_TIB parameter; depressurize input
function [intake, outtake,inside_deadzone_1] = fcn(control, inside_deadzone, PAMs_on,System_on, deadzone_in_TIB, deadzone_out_TIB, depressurize)

[intake, outtake,inside_deadzone_1] = Solenoid(control, inside_deadzone, deadzone_in_TIB, deadzone_out_TIB,PAMs_on,System_on,depressurize);
    
  
end

== matlab function EPA_Walker/PAMs/PAMs Left/SOL/Solenoids ==
  data: control input; intake output; inside_deadzone input; outtake output; inside_deadzone_1 output; deadzone_in input; deadzone_out input; PAMs_on input; System_on input; depressurize input
function [intake, outtake,inside_deadzone_1] = fcn(control, inside_deadzone, deadzone_in, deadzone_out,PAMs_on,System_on,depressurize)

[intake, outtake,inside_deadzone_1] = Solenoid(control, inside_deadzone, deadzone_in, deadzone_out,PAMs_on,System_on,depressurize);
    
  
end

== matlab function EPA_Walker/PAMs/PAMs Left/GAS/Solenoids ==
  data: control input; intake output; inside_deadzone input; outtake output; inside_deadzone_1 output; deadzone_in input; deadzone_out input; PAMs_on input; System_on input; depressurize input
function [intake, outtake,inside_deadzone_1] = fcn(control, inside_deadzone, deadzone_in, deadzone_out,PAMs_on,System_on,depressurize)

[intake, outtake,inside_deadzone_1] = Solenoid(control, inside_deadzone, deadzone_in, deadzone_out,PAMs_on,System_on,depressurize);
    
  
end

== matlab function EPA_Walker/PAMs/PAMs Left/VAS/Solenoids ==
  data: control input; intake output; inside_deadzone input; outtake output; inside_deadzone_1 output; deadzone_in input; deadzone_out input; PAMs_on input; System_on input; depressurize input
function [intake, outtake,inside_deadzone_1] = fcn(control, inside_deadzone, deadzone_in, deadzone_out,PAMs_on,System_on,depressurize)

[intake, outtake,inside_deadzone_1] = Solenoid(control, inside_deadzone, deadzone_in, deadzone_out,PAMs_on,System_on,depressurize);
    
  
end

== matlab function EPA_Walker/PAMs/PAMs Left/POP/Solenoids ==
  data: control input; intake output; inside_deadzone input; outtake output; inside_deadzone_1 output; deadzone_in input; deadzone_out input; PAMs_on input; System_on input; depressurize input
function [intake, outtake,inside_deadzone_1] = fcn(control, inside_deadzone, deadzone_in, deadzone_out,PAMs_on,System_on,depressurize)

[intake, outtake,inside_deadzone_1] = Solenoid(control, inside_deadzone, deadzone_in, deadzone_out,PAMs_on,System_on,depressurize);
    
  
end

== matlab function EPA_Walker/PAMs/PAMs Left/RF/Solenoids ==
  data: control input; intake output; inside_deadzone input; outtake output; inside_deadzone_1 output; deadzone_in input; deadzone_out input; PAMs_on input; System_on input; depressurize input
function [intake, outtake,inside_deadzone_1] = fcn(control, inside_deadzone, deadzone_in, deadzone_out,PAMs_on,System_on,depressurize)

[intake, outtake,inside_deadzone_1] = Solenoid(control, inside_deadzone, deadzone_in, deadzone_out,PAMs_on,System_on,depressurize);
    
  
end

== matlab function EPA_Walker/PAMs/PAMs Left/HAM/Solenoids ==
  data: control input; intake output; inside_deadzone input; outtake output; inside_deadzone_1 output; deadzone_in input; deadzone_out input; PAMs_on input; System_on input; depressurize input
function [intake, outtake,inside_deadzone_1] = fcn(control, inside_deadzone, deadzone_in, deadzone_out,PAMs_on,System_on,depressurize)

[intake, outtake,inside_deadzone_1] = Solenoid(control, inside_deadzone, deadzone_in, deadzone_out,PAMs_on,System_on,depressurize);
    
  
end

== matlab function EPA_Walker/PAMs/PAMs Left/IL/Solenoids ==
  data: control input; intake output; inside_deadzone input; outtake output; inside_deadzone_1 output; deadzone_in input; deadzone_out input; PAMs_on input; System_on input; depressurize input
function [intake, outtake,inside_deadzone_1] = fcn(control, inside_deadzone, deadzone_in, deadzone_out,PAMs_on,System_on,depressurize)

[intake, outtake,inside_deadzone_1] = Solenoid(control, inside_deadzone, deadzone_in, deadzone_out,PAMs_on,System_on,depressurize);
    
  
end

== matlab function EPA_Walker/PAMs/PAMs Left/GL/Solenoids ==
  data: control input; intake output; inside_deadzone input; outtake output; inside_deadzone_1 output; deadzone_in input; deadzone_out input; PAMs_on input; System_on input; depressurize input
function [intake, outtake,inside_deadzone_1] = fcn(control, inside_deadzone, deadzone_in, deadzone_out,PAMs_on,System_on,depressurize)

[intake, outtake,inside_deadzone_1] = Solenoid(control, inside_deadzone, deadzone_in, deadzone_out,PAMs_on,System_on,depressurize);
    
  
end

== matlab function EPA_Walker/Ethernet Communication/Inputs/GRF Slave/GRFz /Hip Position Transformation ==
  data: x_int input; GRF_z output; GRF_MIN parameter; GRF_MAX parameter; bits_GRF parameter
function GRF_z = uint_to_float(x_int, GRF_MIN, GRF_MAX, bits_GRF)
    GRF_z = uint_to_float(x_int, GRF_MIN, GRF_MAX, bits_GRF);
end

== matlab function EPA_Walker/Ethernet Communication/Inputs/GRF Slave/GRFy /Hip Position Transformation ==
  data: x_int input; GRF_y output; GRF_MIN parameter; GRF_MAX parameter; bits_GRF parameter
function GRF_y = uint_to_float(x_int, GRF_MIN, GRF_MAX, bits_GRF)
    GRF_y = uint_to_float(x_int, GRF_MIN, GRF_MAX, bits_GRF);
end

== matlab function EPA_Walker/Ethernet Communication/Inputs/GRF Slave/GRFx /Hip Position Transformation ==
  data: x_int input; GRF_x output; GRF_MIN parameter; GRF_MAX parameter; bits_GRF parameter
function GRF_x = uint_to_float(x_int, GRF_MIN, GRF_MAX, bits_GRF)
    GRF_x = uint_to_float(x_int, GRF_MIN, GRF_MAX, bits_GRF);
end

== matlab function EPA_Walker/Ethernet Communication/Inputs/Motor Right/Byte Splitting Hip ==
  data: byte input; Vel_low output; Curr_h output
function [Vel_low,Curr_h] = fcn(byte)

Vel_low = bitshift(byte,-4);
Curr_h = bitand(byte,15);

== matlab function EPA_Walker/Ethernet Communication/Inputs/Motor Right/Byte Splitting Knee ==
  data: byte input; Vel_low output; Curr_h output
function [Vel_low,Curr_h] = fcn(byte)

Vel_low = bitshift(byte,-4);
Curr_h = bitand(byte,15);

== matlab function EPA_Walker/Ethernet Communication/Inputs/Motor Right/Hip Current Transformation ==
  data: x_int input; Hip_current output; T_MIN parameter; T_MAX parameter; bits_current parameter
function Hip_current = uint_to_float(x_int, T_MIN, T_MAX, bits_current)
    % Converts an unsigned int to float, given range and number of bits %
    Hip_current = uint_to_float(x_int, T_MIN, T_MAX, bits_current);
end

== matlab function EPA_Walker/Ethernet Communication/Inputs/Motor Right/Hip Position Transformation ==
  data: x_int input; Hip_position output; P_MIN parameter; P_MAX parameter; bits_position parameter
function Hip_position = uint_to_float(x_int, P_MIN, P_MAX, bits_position)
    Hip_position = uint_to_float(x_int, P_MIN, P_MAX, bits_position);
end

== matlab function EPA_Walker/Ethernet Communication/Inputs/Motor Right/Hip Velocity Transformation ==
  data: x_int input; Hip_velocity output; V_MIN parameter; V_MAX parameter; bits_velocity parameter
function Hip_velocity = uint_to_float(x_int, V_MIN, V_MAX, bits_velocity)
    % Converts an unsigned int to float, given range and number of bits %
    Hip_velocity = uint_to_float(x_int, V_MIN, V_MAX, bits_velocity);

end

== matlab function EPA_Walker/Ethernet Communication/Inputs/Motor Right/Knee Current Tranformation ==
  data: x_int input; Knee_current output; T_MIN parameter; T_MAX parameter; bits_current parameter
function Knee_current = uint_to_float(x_int, T_MIN, T_MAX, bits_current)
    Knee_current = uint_to_float(x_int, T_MIN, T_MAX, bits_current);
end

== matlab function EPA_Walker/Ethernet Communication/Inputs/Motor Right/Knee Position Transformation1 ==
  data: x_int input; Knee_position output; P_MIN parameter; P_MAX parameter; bits_position parameter
function Knee_position = uint_to_float(x_int, P_MIN, P_MAX, bits_position)
    Knee_position = uint_to_float(x_int, P_MIN, P_MAX, bits_position);
end

== matlab function EPA_Walker/Ethernet Communication/Inputs/Motor Right/Knee Velocity Transformation1 ==
  data: x_int input; Knee_velocity output; V_MIN parameter; V_MAX parameter; bits_velocity parameter
function Knee_velocity = uint_to_float(x_int, V_MIN, V_MAX, bits_velocity)
    Knee_velocity = uint_to_float(x_int, V_MIN, V_MAX, bits_velocity);
end

== matlab function EPA_Walker/Ethernet Communication/Inputs/PAMs Right/MATLAB Function ==
  data: sensorValue input; pressure output; voltageMultiplier_TIB parameter; voltageBias_TIB parameter; ReadingVoltage parameter; VoltageResolution parameter
function pressure   = fcn(sensorValue,voltageMultiplier_TIB, voltageBias_TIB,ReadingVoltage, VoltageResolution)
pressure   = PressureSensor(sensorValue,voltageMultiplier_TIB, voltageBias_TIB,ReadingVoltage,VoltageResolution);
end

== matlab function EPA_Walker/Ethernet Communication/Inputs/PAMs Right/MATLAB Function1 ==
  data: sensorValue input; pressure output; voltageMultiplier_SOL parameter; voltageBias_SOL parameter; ReadingVoltage parameter; VoltageResolution parameter
function pressure   = fcn(sensorValue,voltageMultiplier_SOL, voltageBias_SOL,ReadingVoltage, VoltageResolution)
pressure   = PressureSensor(sensorValue,voltageMultiplier_SOL, voltageBias_SOL,ReadingVoltage,VoltageResolution);
end

== matlab function EPA_Walker/Ethernet Communication/Inputs/PAMs Right/MATLAB Function2 ==
  data: sensorValue input; pressure output; voltageMultiplier_GAS parameter; voltageBias_GAS parameter; ReadingVoltage parameter; VoltageResolution parameter
function pressure   = fcn(sensorValue,voltageMultiplier_GAS, voltageBias_GAS,ReadingVoltage, VoltageResolution)
pressure   = PressureSensor(sensorValue,voltageMultiplier_GAS, voltageBias_GAS,ReadingVoltage,VoltageResolution);
end

== matlab function EPA_Walker/Ethernet Communication/Inputs/PAMs Right/MATLAB Function3 ==
  data: sensorValue input; pressure output; voltageMultiplier_VAS parameter; voltageBias_VAS parameter; ReadingVoltage parameter; VoltageResolution parameter
function pressure   = fcn(sensorValue,voltageMultiplier_VAS, voltageBias_VAS,ReadingVoltage, VoltageResolution)
pressure   = PressureSensor(sensorValue,voltageMultiplier_VAS, voltageBias_VAS,ReadingVoltage,VoltageResolution);
end

== matlab function EPA_Walker/Ethernet Communication/Inputs/PAMs Right/MATLAB Function4 ==
  data: sensorValue input; pressure output; voltageMultiplier_POP parameter; voltageBias_POP parameter; ReadingVoltage parameter; VoltageResolution parameter
function pressure   = fcn(sensorValue,voltageMultiplier_POP, voltageBias_POP,ReadingVoltage, VoltageResolution)
pressure   = PressureSensor(sensorValue,voltageMultiplier_POP, voltageBias_POP,ReadingVoltage,VoltageResolution);
end

== matlab function EPA_Walker/Ethernet Communication/Inputs/PAMs Right/MATLAB Function5 ==
  data: sensorValue input; pressure output; voltageMultiplier_RF parameter; voltageBias_RF parameter; ReadingVoltage parameter; VoltageResolution parameter
function pressure   = fcn(sensorValue,voltageMultiplier_RF, voltageBias_RF,ReadingVoltage, VoltageResolution)
pressure   = PressureSensor(sensorValue,voltageMultiplier_RF, voltageBias_RF,ReadingVoltage,VoltageResolution);
end
